simulink model "tpp_config_interrupt_read_write_register"  (Simulink 9.0)
settings: Solver=FixedStepDiscrete  StartTime=0.0  StopTime=10.0  FixedStep=0.01  RelTol=1e-3
InitFcn:
  | mbd_s32k_consistency_checks(bdroot(gcs));
undefined symbols (not defined in the file): LQFP
libraries: mbd_msd_ec_toolbox x7, mbd_s32k1xx_ec_toolbox x6, simulink x1
Description:
  | This model demonstrates how to use Config, Interrupt, Read and Write Register blocks of TPP.
  | Initially TPP is enabled and it has interrupt enabled. With an oscilloscope, on PHA, PHB, PHC it can be seen PWM signals.
  | 
  | !!!Warnings :
  | -please disconect any load from outputs of DEVKIT-MOTORGD (eg.: coil, motor, low value resistor)
  | - it is recommended to test this model using power source with overcurrent protection set to on (@2-3Amps)  for DEVKIT-MOTORGD
  | 
  | Validation:
  | - GREEN Led sould be on (that indicates TPP hasn't generate any interrupt yet),
  | -  open Freemaster project "tpp_config_interrupt_read_write_register.pmp" and watch "Interrupt", "Button" and "reg" variables. All of them must be equal to 0.
  | - With an oscilloscope monitor PHA, PHB, PHC and interrupt pin (PTE10 in this case). Interrupt pin must be LOW and PHx signals must be like in photos.
  | - with a short wire make a short circuit (for a short period of time) between PHB and PHC,
  | - the GREEN led will be off, the interrupt pin (PTE10) will be HIGH and the outputs PHA, PHB, PHC will be disabled,
  | - in freemaster project "Interrupt" will be equal to 1, and "reg" 10 (bit nr. 1 = 1 indicates desaturation event and bit nr. 3 = 1 indicates overcurrent event),
  | - by pressing the SW3 button, the interupt will be cleared, variable "Button" will be equal to 1, and PHA, PHB, and PHC outputs will be on.
  | 
  | HW prerequisite:
  | - S32K144EVB-Q100
  | - DEVKIT-MOTORGD (connected to S32K144EVB-Q100),
  | - an oscilloscopeor logic analyzer,
  | - One Power Adapter 12V (connected to DEVKIT-MOTORGD).
settings Model: Creator=NXP MBDT Team  LastModifiedBy=nxf40284
settings DataIOCC: ExternalInput=off  InitialState=off  SaveFormat=Dataset  SaveOutput=off  SignalLogging=off  SaveTime=off  ReturnWorkspaceOutputs=on
settings OptimizationCC: DefaultParameterBehavior=Inlined  EnhancedBackFolding=on  PassReuseOutputArgsAs=Individual arguments  LifeSpan=auto  OptimizeBlockOrder=speed  DifferentSizesBufferReuse=on
settings DebuggingCC: UnderspecifiedInitializationDetection=Simplified  MergeDetectMultiDrivingBlocksExec=error  InheritedTsInSrcMsg=none  SingleTaskRateTransMsg=error  ParameterTunabilityLossMsg=error  UnconnectedInputMsg=error  UnconnectedOutputMsg=error  UnconnectedLineMsg=error  UnknownTsInhSupMsg=error  SFUnexpectedBacktrackingDiag=error  SFNoUnconditionalDefaultTransitionDiag=error  SFExecutionAtInitializationDiag=warning
settings HardwareCC: ProdLargestAtomicInteger=Long  ProdLargestAtomicFloat=Double  ProdIntDivRoundTo=Zero  ProdEndianess=LittleEndian  ProdHWDeviceType=ARM Compatible->ARM Cortex
settings ModelReferenceCC: PropagateSignalLabelsOutOfModel=on
settings SFSimCC: SimUseLocalCustomCode=on  MATLABDynamicMemAlloc=off
settings RTWCC: SystemTargetFile=mbd_s32k.tlc  MakeCommand=mbd_s32k_make_rtw COPY_MDLREF_INCLUDES=0  TemplateMakefile=mbd_s32k.tmf  Description=Model Based Design Toolbox S32K14x Code Generation Target  GenerateReport=on  RTWUseLocalCustomCode=on  IncludeHyperlinkInReport=on  LaunchReport=on  GenerateTraceInfo=on  GenerateTraceReport=on  GenerateTraceReportSl=on  GenerateTraceReportSf=on  GenerateTraceReportEml=on
settings CodeAppCC: ForceParamTrailComments=on  IgnoreCustomStorageClasses=off  OperatorAnnotations=on  SimulinkDataObjDesc=on  SFDataObjDesc=on  InsertBlockDesc=on  StateflowObjectComments=off
settings STFCustomTargetCC: TargetLangStandard=C99 (ISO)  MultiwordLength=256  CombineOutputUpdateFcns=on  ERTCustomFileBanners=on  SupportContinuousTime=off  SupportNonInlinedSFcns=off  RemoveResetFunc=on  MATLABClassNameForMDSCustomization=Simulink.SoftwareTarget.ERTCustomization  GRTInterface=off  SystemTargetFile=mbd_s32k.tlc
settings ERTTargetCC: TargetLangStandard=C99 (ISO)  ParMdlRefBuildCompliant=off  CompOptLevelCompliant=off  ConcurrentExecutionCompliant=off  ModelStepFunctionPrototypeControlCompliant=off  CPPClassGenCompliant=off  UseToolchainInfoCompliant=off  InlinedParameterPlacement=NonHierarchical  ERTSrcFileBannerTemplate=mbd_ert_code_template.cgt  ERTHdrFileBannerTemplate=mbd_ert_code_template.cgt  ERTDataSrcFileTemplate=mbd_ert_code_template.cgt  ERTDataHdrFileTemplate=mbd_ert_code_template.cgt  ERTCustomFileTemplate=example_file_process.tlc
settings ConfigComp: CovMetricSettings=dwe  CovHtmlReporting=off  CovSaveCumulativeToWorkspaceVar=off  CovSaveSingleToWorkspaceVar=off  CovExternalEMLEnable=on

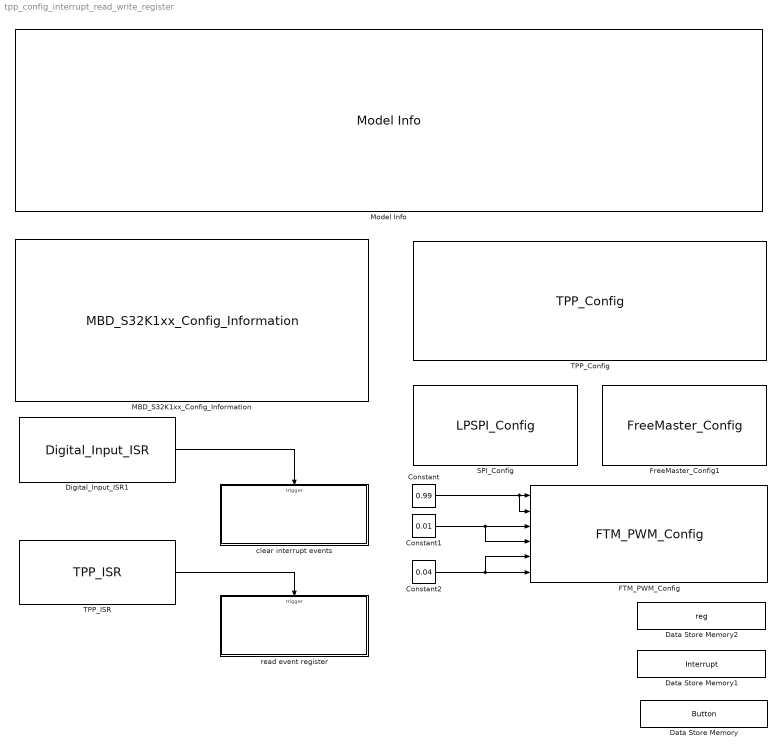
== system tpp_config_interrupt_read_write_register ==
  Constant : Constant  Value=0.99  OutDataTypeStr=single
  Constant1 : Constant  Value=0.01  OutDataTypeStr=single
  Constant2 : Constant  Value=0.04  OutDataTypeStr=single
  Data Store Memory : DataStoreMemory  DataStoreName=Button  ReadBeforeWriteMsg=warning  WriteAfterWriteMsg=warning  WriteAfterReadMsg=warning  ShowAdditionalParam=off  OutDataTypeStr=boolean
  Data Store Memory1 : DataStoreMemory  DataStoreName=Interrupt  ReadBeforeWriteMsg=warning  WriteAfterWriteMsg=warning  WriteAfterReadMsg=warning  ShowAdditionalParam=off  OutDataTypeStr=boolean
  Data Store Memory2 : DataStoreMemory  DataStoreName=reg  ReadBeforeWriteMsg=warning  WriteAfterWriteMsg=warning  WriteAfterReadMsg=warning  ShowAdditionalParam=off  OutDataTypeStr=uint8
  Digital_Input_ISR1 : mbd_s32k1xx_ec_toolbox/GPIO Blocks/Digital_Input_ISR  gpio_pin=PTC13: [PTC13 | Port C I/O]  irqc=on falling-edge  prio=15
  FTM_PWM_Config : mbd_s32k1xx_ec_toolbox/Motor Control Blocks/FTM Blocks/FTM_PWM_Config  ftmModule=3  ftmMode=Center-Aligned PWM  ftmSourceClock=80 MHz  swcontrol_enable=off  chan0En=on  chan0Type=Independent  chan2En=on  chan2Type=Independent  chan4En=on  chan4Type=Independent  chan6En=off  chan6Type=Independent  ftmPwmUnits=Hz  outFrequency=20000  ftmPeriod=4000  ftmPrescaler=Divide by 1  deadtimeUnits=Nanoseconds  deadtimeNs=0  deadtimeTicks=0  deadtimePrescaler=Divide by 1  dutyCycleCh0=0.002  dutyCycleCh1=0.002  dutyCycleCh2=0.002  dutyCycleCh3=0.002  dutyCycleCh4=0.002  dutyCycleCh5=0.002  dutyCycleCh6=0.25  dutyCycleCh7=0.25  dutyCycleSim=off  startAfterInit=on  showAdvOpt=on  pinFtmCh0=PTB8: [FTM3_CH0 | FTM Channel]  pinFtmCh1=PTB9: [FTM3_CH1 | FTM Channel]  pinPolCh0=Active Low  pinPolCh1=Active Low  outputComplem0=Main inverted  outputLevel0=Low  outputLevel1=Low  pinFtmCh2=PTB10: [FTM3_CH2 | FTM Channel]  pinFtmCh3=PTB11: [FTM3_CH3 | FTM Channel]  pinPolCh2=Active High  pinPolCh3=Active High  outputComplem2=Main inverted  outputLevel2=Low  outputLevel3=Low  pinFtmCh4=PTC10: [FTM3_CH4 | FTM Channel]  pinFtmCh5=PTC11: [FTM3_CH5 | FTM Channel]  pinPolCh4=Active Low  pinPolCh5=Active Low  outputComplem4=Main inverted  outputLevel4=Low  outputLevel5=Low  pinFtmCh6=PTC12: [FTM3_CH6 | FTM Channel]  pinFtmCh7=None  pinPolCh6=Active Low  pinPolCh7=Active Low  outputComplem6=Main duplicated  outputLevel6=Low  outputLevel7=Low  initTrigger=off  chTrigger0=off  chTrigger1=off  chTrigger2=off  chTrigger3=off  chTrigger4=off  chTrigger5=off  chTrigger6=off  chTrigger7=off  mcuTargetUpdate=on  pwmSyncTrg=Software trigger  pwmSyncHwRouting=TRGMUX_FTM7  pwmSyncTrg0=off  pwmSyncTrg1=off  pwmSyncTrg2=off  pwmSyncAutoClear=on  pwmSyncMinLoad=on  pwmSyncMaxLoad=on  pwmSyncInvert=System Clock  pwmSyncOutControl=System Clock  pwmSyncOutMask=System Clock  pwmSyncCounterInitial=System Clock  pwmSyncPoints=Update now  reloadEnable=off  reloadPriority=15  reloadHalfCycle=off  reloadHCR=0  reloadFrequency=0  chnMatch0=off  chnMatch1=off  chnMatch2=off  chnMatch3=off  chnMatch4=off  chnMatch5=off  chnMatch6=off  chnMatch7=off  pwmFaultProtection=off  pwmFaultInterrupt=off  pwmFaultClearing=Fault control disabled  pwmFaultPinState=Safe Value  pwmFaultFilterValue=0  pwmFaultPriority=15  fault_disen_0=off  fault_filter_0=off  fault_polarity_0=Active High  fault_disen_1=off  fault_filter_1=off  fault_polarity_1=Active high  fault_disen_2=off  fault_filter_2=off  fault_polarity_2=Active high  fault_disen_3=off  fault_filter_3=off  fault_polarity_3=Active high  fault_pin_0=None  fault_pin_1=None  fault_pin_2=None  fault_pin_3=None
  FreeMaster_Config1 : mbd_s32k1xx_ec_toolbox/Utility Blocks/FreeMaster_Config  interface=LPUART1  baudrate=115200  rxd=PTC6: [LPUART1_RX | Receive]  txd=PTC7: [LPUART1_TX | Transmit]  mode=Short Interrupt  isr_prio=15  show_adv_opts=on  use_scope=on  max_scope_vars=8  use_recorder=on  max_rec_vars=8  rec_buff_size=1024  rec_timebase=0 seconds  comm_buffer_size_auto=on  comm_buffer_size=255  comm_rqueue_size_default=on  comm_rqueue_size=32
  MBD_S32K1xx_Config_Information : mbd_s32k1xx_ec_toolbox/MBD_S32K1xx_Config_Information  mbdt_ver=0  disp_str=|  config_params=[]  mcu_target_name=S32K144  mcu_target_package=100-LQFP  mcu_target_sram_size=64KB  mcu_system_clock_freq=80  mcu_xtal_freq=External 8  mcu_steptick_timer=LPIT Channel 0  mcu_steptick_prio=15  ds_import_enable=on  target_compiler=GCC  target_memory=FLASH  gcc_target_compile_opts=-mcpu=cortex-m4 -mthumb -mfloat-abi=hard -mfpu=fpv4-sp-d16 -O1 -g -gstrict-dwarf  gcc_target_assemble_opts=-mcpu=cortex-m4 -mthumb -mfloat-abi=hard -mfpu=fpv4-sp-d16 -g  gcc_target_link_opts=-mcpu=cortex-m4 -mthumb -mfloat-abi=hard -mfpu=fpv4-sp-d16  gcc_target_default_lcf=on  gcc_target_user_lcf=S32K144_64_flash.ld  ghs_target_compile_opts=-cpu=cortexm4f -thumb -DARM_MATH_CM4 -fpu=vfpv4_d16 -fsingle -Ogeneral -Wundef -Wimplicit-int -Wshadow -Wtrigraphs --no_commons --gnu_asm -gnu99 -gdwarf-2 -G  ghs_target_assemble_opts=-cpu=cortexm4f -fpu=vfpv4_d16  ghs_target_link_opts=-cpu=cortexm4f -thumb -fpu=vfpv4_d16  ghs_target_default_lcf=on  ghs_target_user_lcf=S32K144_64_flash.ld  iar_target_compile_opts=--cpu=Cortex-M4F --thumb --fpu=VFPv4_sp -Ol -e --debug --dlib_config normal  iar_target_assemble_opts=--cpu Cortex-M4F --thumb --fpu VFPv4_sp  iar_target_link_opts=--no_exceptions --vfe --inline  iar_target_default_lcf=on  iar_target_user_lcf=S32K144_64_flash.icf  pil_download_enable=off  rbl_download_enable=on  rbl_start_delay=5000  rbl_download_interface=OpenSDA  rbl_restart_request=off  rbl_com_port=Custom  rbl_com_port_custom=COM1  pil_download_rate=57600  pil_opensda_drive=Custom  pil_opensda_drive_custom=D  pil_uart_instance=0  pil_uart_rx=PTA2: [LPUART0_RX | Receive]  pil_uart_tx=PTA3: [LPUART0_TX | Transmit]  FTM_PWM_PcrCheckEnDis=on  FTM_Input_Edge_Inputs_PcrCheckEnDis=on  FTM_Dual_Edge_Inputs_PcrCheckEnDis=on  FTM_Quadrature_Inputs_PcrCheckEnDis=on  FTM_Hall_Sensor_Inputs_PcrCheckEnDis=on  LPTMR_PcrCheckEnDis=on  PIT_PcrCheckEnDis=on  RTC_PcrCheckEnDis=on  FlexCAN_PcrCheckEnDis=on  LIN_PcrCheckEnDis=on  FlexIO_PcrCheckEnDis=on  LPI2C_PcrCheckEnDis=on  LPSPI_PcrCheckEnDis=on  LPUART_PcrCheckEnDis=on  CMP_PcrCheckEnDis=on  GPIO_OutputPcrCheckEnDis=on  GPIO_InputPcrCheckEnDis=on  SBC_PcrCheckEnDis=on  AMMCLIB_PcrCheckEnDis=on  FM_PcrCheckEnDis=on  Profile_PcrCheckEnDis=on  ConfigParams_PcrCheckEnDis=on  ModelRef_PcrCheckEnDis=on  PDB0_PcrCheckEnDis=on  CSEc_PcrCheckEnDis=on  eDMA_PcrCheckEnDis=on  ADC_PcrCheckEnDis=on  WDOG_PcrCheckEnDis=on
      | Target : S32K144-64KB_SRAM
      | Package : 100-pin
      | System clock : 80 MHz
      | XTAL clock : External 8 MHz
      | Compiler : IAR
      | Target Type : FLASH
      | Download Code after build : off
      | Step Tick Interrupt Priority : 15
  Model Info : simulink/Model-Wide Utilities/Model Info  Frame=on  DisplayStringWithTags=|  HorizontalTextAlignment=Left  LeftAlignmentValue=0.02
      | Model Name: %<ModelName>
      | 
      | Description: %<Description>
  "SPI_Config " : mbd_s32k1xx_ec_toolbox/Communication Blocks/SPI Blocks/LPSPI_Config   Priority=2  InstanceNumber=0  Role=Master  BaudRate=500000  ShowAdvanced=on  sin=PTB3: [LPSPI0_SIN | LPSPI Serial Data Input]  sout=PTB4: [LPSPI0_SOUT | LPSPI Serial Data Output]  sck=PTB2: [LPSPI0_SCK | LPSPI Serial Clock I/O]  pcs0=None  pcs1=None  pcs2=None  pcs3=None  CPHA=1  CPOL=0  BitOrder=MSB first  TransferSize=8  WhichPCS=0  PCSPol=ActiveHigh  ContinuousTransfer=off
  TPP_Config : mbd_msd_ec_toolbox/TPP/TPP_Config  Priority=1  tppInstance=0  desatMode=off  fullonMode=off  lockMode=off  overtempEvent=on  phaseEvent=on  desatEvent=on  framingEvent=on  vlsEvent=on  writeErrEvent=on  overcurrentEvent=on  resetEvent=on  mcuTppIntEn=on  prioInt=15  tppDeadtime=200  initTppNow=on  tppSpiInst=Please add SPI block to workspace  tppPwmModule=Please add FTM block to workspace  tppPair0_1=on  tppPair2_3=on  tppPair4_5=on  tppPair6_7=off  tppFirstChHS=on  tppEn1Pin=PTA2: [PTA2 | Port A I/O]  tppEn2Pin=PTA2: [PTA2 | Port A I/O]  tppRstPin=PTA3: [PTA3 | Port A I/O]  tppCsPin=PTB5: [PTB5 | Port B I/O]  tppIntPin=PTE10: [PTE10 | Port E I/O]
  TPP_ISR : mbd_msd_ec_toolbox/TPP/TPP_ISR  tppInstance=0
  clear interrupt events : Subsystem
  read event register : Subsystem  TreatAsAtomicUnit=on
  wires:
  TPP_ISR/1 -> read event register/Trigger
  Constant/1 -> FTM_PWM_Config/2, FTM_PWM_Config/1
  Digital_Input_ISR1/1 -> clear interrupt events/Trigger
  Constant1/1 -> FTM_PWM_Config/4, FTM_PWM_Config/3
  Constant2/1 -> FTM_PWM_Config/5, FTM_PWM_Config/6

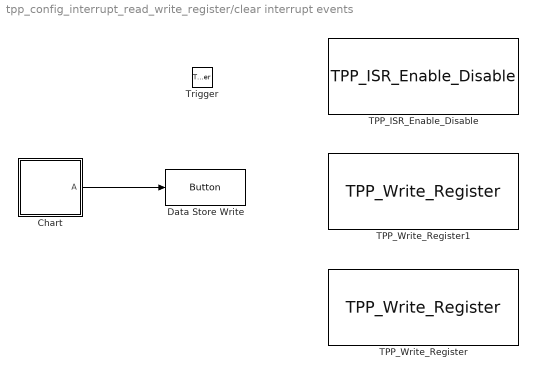
== system tpp_config_interrupt_read_write_register/clear interrupt events ==
  Trigger : TriggerPort  TriggerType=function-call  VariantControl=Variant  PortDimensions=1
  Chart : Stateflow chart  TreatAsAtomicUnit=on
  Data Store Write : DataStoreWrite  DataStoreName=Button
  TPP_ISR_Enable_Disable : mbd_msd_ec_toolbox/TPP/TPP_ISR_Enable_Disable  Priority=4  tppInstance=0  mcuTppIntEn=on  prioInt=15
  TPP_Write_Register : mbd_msd_ec_toolbox/TPP/TPP_Write_Register  tppInstance=0  tppRegister=TPP_CLINT1  lockMode=on  tppMode_b4=off  fullonMode=on  tppMode_b5=off  tppMode_b2=off  tppMode_b6=on  desatMode=on  tppMode_b7=off  clearPhaseEvent=on  tppClint1b4=on  clearFramingEvent=on  tppClint1b5=on  clearWriteErrEvent=on  tppClint1b6=on  clearResetEvent=on  tppClint1b7=off  clearOvertempEvent=on  tppClint0b4=off  clearDesatEvent=on  tppClint0b5=on  clearVlsEvent=on  tppClint0b6=on  clearOvercurrentEvent=on  tppClint0b7=off  overtempEvent=off  tppMask0b4=off  desatEvent=off  tppMask0b5=on  vlsEvent=off  tppMask0b6=off  overcurrentEvent=off  tppMask0b7=off  phaseEvent=on  tppMask1b4=on  framingEvent=on  tppMask1b5=on  writeErrEvent=on  tppMask1b6=off  resetEvent=on  tppMask1b7=off
  TPP_Write_Register1 : mbd_msd_ec_toolbox/TPP/TPP_Write_Register  tppInstance=0  tppRegister=TPP_CLINT0  lockMode=on  tppMode_b4=off  fullonMode=on  tppMode_b5=off  tppMode_b2=off  tppMode_b6=on  desatMode=on  tppMode_b7=off  clearPhaseEvent=on  tppClint1b4=on  clearFramingEvent=on  tppClint1b5=on  clearWriteErrEvent=on  tppClint1b6=on  clearResetEvent=on  tppClint1b7=off  clearOvertempEvent=on  tppClint0b4=off  clearDesatEvent=on  tppClint0b5=on  clearVlsEvent=on  tppClint0b6=on  clearOvercurrentEvent=on  tppClint0b7=off  overtempEvent=off  tppMask0b4=off  desatEvent=off  tppMask0b5=on  vlsEvent=off  tppMask0b6=off  overcurrentEvent=off  tppMask0b7=off  phaseEvent=on  tppMask1b4=on  framingEvent=on  tppMask1b5=on  writeErrEvent=on  tppMask1b6=off  resetEvent=on  tppMask1b7=off
  wires:
  Chart/1(" A") -> Data Store Write/1

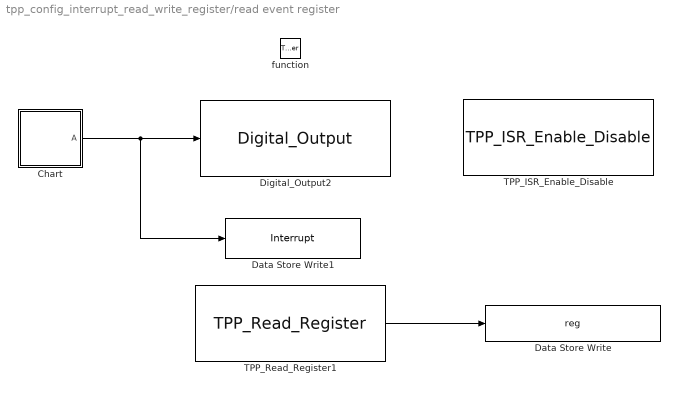
== system tpp_config_interrupt_read_write_register/read event register ==
  function : TriggerPort  TriggerType=function-call  VariantControl=Variant
  Chart : Stateflow chart  TreatAsAtomicUnit=on
  Data Store Write : DataStoreWrite  DataStoreName=reg
  Data Store Write1 : DataStoreWrite  DataStoreName=Interrupt
  Digital_Output2 : mbd_s32k1xx_ec_toolbox/GPIO Blocks/Digital_Output  gpio_pin=PTD16: [PTD16 | Port D I/O]  init_val=Low  drive_strength=Low
  TPP_ISR_Enable_Disable : mbd_msd_ec_toolbox/TPP/TPP_ISR_Enable_Disable  Priority=4  tppInstance=0  mcuTppIntEn=off  prioInt=15
  TPP_Read_Register1 : mbd_msd_ec_toolbox/TPP/TPP_Read_Register  tppInstance=0  tppRegister=TPP_Status_Register_0
  wires:
  Chart/1(" A") -> Data Store Write1/1, Digital_Output2/1
  TPP_Read_Register1/1 -> Data Store Write/1

== stateflow chart read event register/Chart ==
  state A
  state A1
  (default) -> A
  A -> A1
  A1 -> A
  data: A output boolean [0..1]

== stateflow chart clear interrupt events/Chart ==
  state A
  state A1
  (default) -> A
  A -> A1
  A1 -> A
  data: A output boolean [0..1]
